simulink model "wind_plant"  (R2025b)
settings: Solver=ode4  StartTime=0.0  StopTime=wind_p.T(2)  FixedStep=wind_p.h  RelTol=1e-3
values from neighbouring files (symbols this model uses):
  wind_p = wind_plant_parameters()    [build_wind_plant.m]
settings Model: Creator=yuexi  LastModifiedBy=yuexi

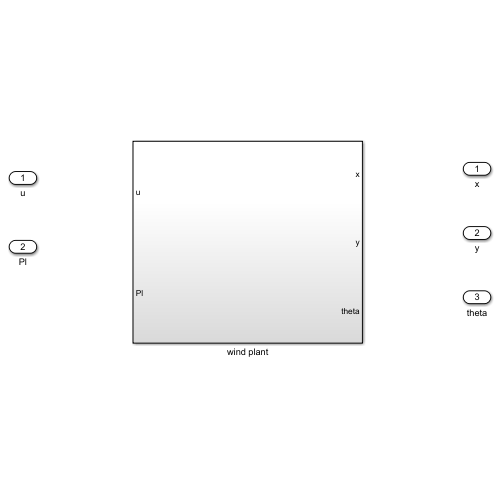
[thumbnail: Simulink's stored preview of the top-level diagram]
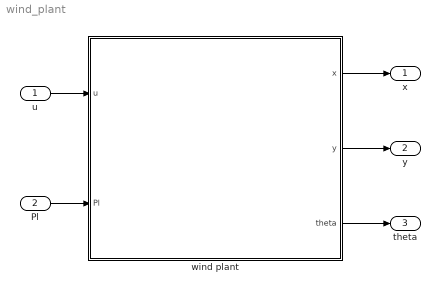
== system wind_plant ==
  u : Inport
  Pl : Inport  Port=2
  wind plant : Subsystem
  x : Outport
  y : Outport  Port=2
  theta : Outport  Port=3
  wires:
  Pl/1 -> wind plant/2(Pl)
  u/1 -> wind plant/1(u)
  wind plant/3(theta) -> theta/1
  wind plant/2(y) -> y/1
  wind plant/1(x) -> x/1

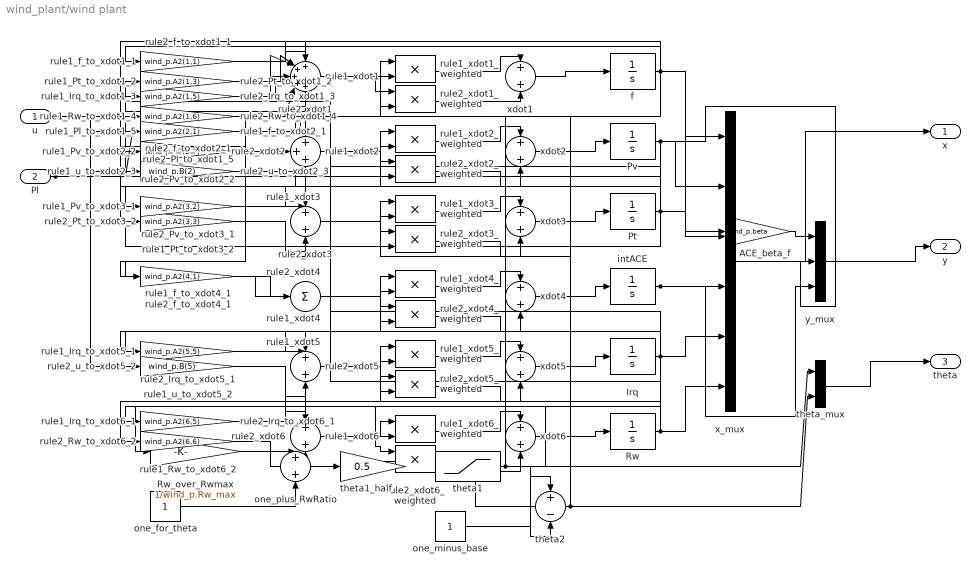
== system wind_plant/wind plant ==
  u : Inport
  Pl : Inport  Port=2
  ACE_beta_f : Gain  Gain=wind_p.beta
  Irq : Integrator  InitialCondition=wind_p.x0(5)
  Pt : Integrator  InitialCondition=wind_p.x0(3)
  Pv : Integrator  InitialCondition=wind_p.x0(2)
  Rw : Integrator  InitialCondition=wind_p.x0(6)
  Rw_over_Rwmax : Gain  Gain=1/wind_p.Rw_max
  f : Integrator  InitialCondition=wind_p.x0(1)
  intACE : Integrator  InitialCondition=wind_p.x0(4)
  one_for_theta : Constant
  one_minus_base : Constant
  one_plus_RwRatio : Sum
  rule1_Irq_to_xdot1_3 : Gain  Gain=wind_p.A1(1,5)
  rule1_Irq_to_xdot5_1 : Gain  Gain=wind_p.A1(5,5)
  rule1_Irq_to_xdot6_1 : Gain  Gain=wind_p.A1(6,5)
  rule1_Pl_to_xdot1_5 : Gain  Gain=wind_p.E(1)
  rule1_Pt_to_xdot1_2 : Gain  Gain=wind_p.A1(1,3)
  rule1_Pt_to_xdot3_2 : Gain  Gain=wind_p.A1(3,3)
  rule1_Pv_to_xdot2_2 : Gain  Gain=wind_p.A1(2,2)
  rule1_Pv_to_xdot3_1 : Gain  Gain=wind_p.A1(3,2)
  rule1_Rw_to_xdot1_4 : Gain  Gain=wind_p.A1(1,6)
  rule1_Rw_to_xdot6_2 : Gain  Gain=wind_p.A1(6,6)
  rule1_f_to_xdot1_1 : Gain  Gain=wind_p.A1(1,1)
  rule1_f_to_xdot2_1 : Gain  Gain=wind_p.A1(2,1)
  rule1_f_to_xdot4_1 : Gain  Gain=wind_p.A1(4,1)
  rule1_u_to_xdot2_3 : Gain  Gain=wind_p.B(2)
  rule1_u_to_xdot5_2 : Gain  Gain=wind_p.B(5)
  rule1_xdot1 : Sum  Inputs=+++++
  rule1_xdot1_weighted : Product
  rule1_xdot2 : Sum  Inputs=+++
  rule1_xdot2_weighted : Product
  rule1_xdot3 : Sum
  rule1_xdot3_weighted : Product
  rule1_xdot4 : Sum  Inputs=+
  rule1_xdot4_weighted : Product
  rule1_xdot5 : Sum
  rule1_xdot5_weighted : Product
  rule1_xdot6 : Sum
  rule1_xdot6_weighted : Product
  rule2_Irq_to_xdot1_3 : Gain  Gain=wind_p.A2(1,5)
  rule2_Irq_to_xdot5_1 : Gain  Gain=wind_p.A2(5,5)
  rule2_Irq_to_xdot6_1 : Gain  Gain=wind_p.A2(6,5)
  rule2_Pl_to_xdot1_5 : Gain  Gain=wind_p.E(1)
  rule2_Pt_to_xdot1_2 : Gain  Gain=wind_p.A2(1,3)
  rule2_Pt_to_xdot3_2 : Gain  Gain=wind_p.A2(3,3)
  rule2_Pv_to_xdot2_2 : Gain  Gain=wind_p.A2(2,2)
  rule2_Pv_to_xdot3_1 : Gain  Gain=wind_p.A2(3,2)
  rule2_Rw_to_xdot1_4 : Gain  Gain=wind_p.A2(1,6)
  rule2_Rw_to_xdot6_2 : Gain  Gain=wind_p.A2(6,6)
  rule2_f_to_xdot1_1 : Gain  Gain=wind_p.A2(1,1)
  rule2_f_to_xdot2_1 : Gain  Gain=wind_p.A2(2,1)
  rule2_f_to_xdot4_1 : Gain  Gain=wind_p.A2(4,1)
  rule2_u_to_xdot2_3 : Gain  Gain=wind_p.B(2)
  rule2_u_to_xdot5_2 : Gain  Gain=wind_p.B(5)
  rule2_xdot1 : Sum  Inputs=+++++
  rule2_xdot1_weighted : Product
  rule2_xdot2 : Sum  Inputs=+++
  rule2_xdot2_weighted : Product
  rule2_xdot3 : Sum
  rule2_xdot3_weighted : Product
  rule2_xdot4 : Sum  Inputs=+
  rule2_xdot4_weighted : Product
  rule2_xdot5 : Sum
  rule2_xdot5_weighted : Product
  rule2_xdot6 : Sum
  rule2_xdot6_weighted : Product
  theta1 : Saturate  UpperLimit=1  LowerLimit=0
  theta1_half : Gain  Gain=0.5
  theta2 : Sum  Inputs=+-
  theta_mux : Mux  Inputs=2
  x_mux : Mux  Inputs=6
  xdot{1..6} (6 alike) : Sum
  y_mux : Mux  Inputs=3
  x : Outport
  y : Outport  Port=2
  theta : Outport  Port=3
  wires:
  f/1 -> x_mux/1, rule1_f_to_xdot1_1/1, rule1_f_to_xdot2_1/1, rule1_f_to_xdot4_1/1, rule2_f_to_xdot1_1/1, rule2_f_to_xdot2_1/1, rule2_f_to_xdot4_1/1, ACE_beta_f/1
  Pv/1 -> x_mux/2, rule1_Pv_to_xdot2_2/1, rule1_Pv_to_xdot3_1/1, rule2_Pv_to_xdot2_2/1, rule2_Pv_to_xdot3_1/1, y_mux/2
  Pt/1 -> x_mux/3, rule1_Pt_to_xdot1_2/1, rule1_Pt_to_xdot3_2/1, rule2_Pt_to_xdot1_2/1, rule2_Pt_to_xdot3_2/1
  intACE/1 -> x_mux/4, y_mux/3
  Irq/1 -> x_mux/5, rule1_Irq_to_xdot1_3/1, rule1_Irq_to_xdot5_1/1, rule1_Irq_to_xdot6_1/1, rule2_Irq_to_xdot1_3/1, rule2_Irq_to_xdot5_1/1, rule2_Irq_to_xdot6_1/1
  Rw/1 -> x_mux/6, Rw_over_Rwmax/1, rule1_Rw_to_xdot1_4/1, rule1_Rw_to_xdot6_2/1, rule2_Rw_to_xdot1_4/1, rule2_Rw_to_xdot6_2/1
  x_mux/1 -> x/1
  Rw_over_Rwmax/1 -> one_plus_RwRatio/1
  one_for_theta/1 -> one_plus_RwRatio/2
  one_plus_RwRatio/1 -> theta1_half/1
  theta1_half/1 -> theta1/1
  one_minus_base/1 -> theta2/1
  theta1/1 -> theta2/2, theta_mux/1, rule1_xdot1_weighted/2, rule1_xdot2_weighted/2, rule1_xdot3_weighted/2, rule1_xdot4_weighted/2, rule1_xdot5_weighted/2, rule1_xdot6_weighted/2
  theta2/1 -> theta_mux/2, rule2_xdot1_weighted/2, rule2_xdot2_weighted/2, rule2_xdot3_weighted/2, rule2_xdot4_weighted/2, rule2_xdot5_weighted/2, rule2_xdot6_weighted/2
  theta_mux/1 -> theta/1
  rule1_f_to_xdot1_1/1 -> rule1_xdot1/1
  rule1_Pt_to_xdot1_2/1 -> rule1_xdot1/2
  rule1_Irq_to_xdot1_3/1 -> rule1_xdot1/3
  rule1_Rw_to_xdot1_4/1 -> rule1_xdot1/4
  Pl/1 -> rule1_Pl_to_xdot1_5/1, rule2_Pl_to_xdot1_5/1
  rule1_Pl_to_xdot1_5/1 -> rule1_xdot1/5
  rule1_f_to_xdot2_1/1 -> rule1_xdot2/1
  rule1_Pv_to_xdot2_2/1 -> rule1_xdot2/2
  u/1 -> rule1_u_to_xdot2_3/1, rule1_u_to_xdot5_2/1, rule2_u_to_xdot2_3/1, rule2_u_to_xdot5_2/1
  rule1_u_to_xdot2_3/1 -> rule1_xdot2/3
  rule1_Pv_to_xdot3_1/1 -> rule1_xdot3/1
  rule1_Pt_to_xdot3_2/1 -> rule1_xdot3/2
  rule1_f_to_xdot4_1/1 -> rule1_xdot4/1
  rule1_Irq_to_xdot5_1/1 -> rule1_xdot5/1
  rule1_u_to_xdot5_2/1 -> rule1_xdot5/2
  rule1_Irq_to_xdot6_1/1 -> rule1_xdot6/1
  rule1_Rw_to_xdot6_2/1 -> rule1_xdot6/2
  rule2_f_to_xdot1_1/1 -> rule2_xdot1/1
  rule2_Pt_to_xdot1_2/1 -> rule2_xdot1/2
  rule2_Irq_to_xdot1_3/1 -> rule2_xdot1/3
  rule2_Rw_to_xdot1_4/1 -> rule2_xdot1/4
  rule2_Pl_to_xdot1_5/1 -> rule2_xdot1/5
  rule2_f_to_xdot2_1/1 -> rule2_xdot2/1
  rule2_Pv_to_xdot2_2/1 -> rule2_xdot2/2
  rule2_u_to_xdot2_3/1 -> rule2_xdot2/3
  rule2_Pv_to_xdot3_1/1 -> rule2_xdot3/1
  rule2_Pt_to_xdot3_2/1 -> rule2_xdot3/2
  rule2_f_to_xdot4_1/1 -> rule2_xdot4/1
  rule2_Irq_to_xdot5_1/1 -> rule2_xdot5/1
  rule2_u_to_xdot5_2/1 -> rule2_xdot5/2
  rule2_Irq_to_xdot6_1/1 -> rule2_xdot6/1
  rule2_Rw_to_xdot6_2/1 -> rule2_xdot6/2
  rule1_xdot1/1 -> rule1_xdot1_weighted/1
  rule2_xdot1/1 -> rule2_xdot1_weighted/1
  rule1_xdot1_weighted/1 -> xdot1/1
  rule2_xdot1_weighted/1 -> xdot1/2
  xdot1/1 -> f/1
  rule1_xdot2/1 -> rule1_xdot2_weighted/1
  rule2_xdot2/1 -> rule2_xdot2_weighted/1
  rule1_xdot2_weighted/1 -> xdot2/1
  rule2_xdot2_weighted/1 -> xdot2/2
  xdot2/1 -> Pv/1
  rule1_xdot3/1 -> rule1_xdot3_weighted/1
  rule2_xdot3/1 -> rule2_xdot3_weighted/1
  rule1_xdot3_weighted/1 -> xdot3/1
  rule2_xdot3_weighted/1 -> xdot3/2
  xdot3/1 -> Pt/1
  rule1_xdot4/1 -> rule1_xdot4_weighted/1
  rule2_xdot4/1 -> rule2_xdot4_weighted/1
  rule1_xdot4_weighted/1 -> xdot4/1
  rule2_xdot4_weighted/1 -> xdot4/2
  xdot4/1 -> intACE/1
  rule1_xdot5/1 -> rule1_xdot5_weighted/1
  rule2_xdot5/1 -> rule2_xdot5_weighted/1
  rule1_xdot5_weighted/1 -> xdot5/1
  rule2_xdot5_weighted/1 -> xdot5/2
  xdot5/1 -> Irq/1
  rule1_xdot6/1 -> rule1_xdot6_weighted/1
  rule2_xdot6/1 -> rule2_xdot6_weighted/1
  rule1_xdot6_weighted/1 -> xdot6/1
  rule2_xdot6_weighted/1 -> xdot6/2
  xdot6/1 -> Rw/1
  ACE_beta_f/1 -> y_mux/1
  y_mux/1 -> y/1
